simulink model "tearthtest"  (R2018b)
settings: Solver=ode45  StartTime=0.0  StopTime=365*24*3600  RelTol=1e-3  EnableMultiTasking=on
settings Model: Creator=drhf  LastModifiedBy=drhf
settings DataIOCC: LimitDataPoints=on  SaveFormat=Array  SignalLoggingSaveFormat=ModelDataLogs
settings OptimizationCC: ExpressionDepthLimit=2147483647  LifeSpan=inf
settings DebuggingCC: UnderspecifiedInitializationDetection=Classic  MergeDetectMultiDrivingBlocksExec=none  SolverPrmCheckMsg=warning  FcnCallInpInsideContextMsg=warning  StateNameClashWarn=warning  SFUnexpectedBacktrackingDiag=warning  SFNoUnconditionalDefaultTransitionDiag=warning  SFExecutionAtInitializationDiag=none
settings HardwareCC: ProdBitPerPointer=32  ProdBitPerSizeT=32  ProdBitPerPtrDiffT=32  ProdLargestAtomicFloat=None  ProdIntDivRoundTo=Undefined  ProdEndianess=Unspecified  ProdWordSize=32  ProdHWDeviceType=32-bit Generic
settings ModelReferenceCC: PropagateSignalLabelsOutOfModel=off
settings SFSimCC: SimUseLocalCustomCode=off
settings RTWCC: RTWUseLocalCustomCode=off
settings CodeAppCC: StateflowObjectComments=on
settings GRTTargetCC: TargetLangStandard=C89/C90 (ANSI)  GeneratePreprocessorConditionals=Disable all  CombineOutputUpdateFcns=off  GRTInterface=on
settings ConfigComp: CovMetricSettings=dw  CovHtmlReporting=on  CovSaveCumulativeToWorkspaceVar=on  CovSaveSingleToWorkspaceVar=on  CovExternalEMLEnable=off

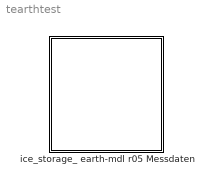
== system tearthtest ==
  ice_storage_ earth-mdl r05 Messdaten : Subsystem  mask(simple water storage){vol=10, l_solar=30*3, l_hp=8*40, f_ice=0.075, t_ini=0, z=3.32-0.12, h=7, dearth=1, Tmeanoutside=11, deltathetae=9.3, Tmeaninside=5, deltathetai=15, tshift=319 %+8760/2 %to get the right behaviour!, cond_ground=5, cp_ground=800, rho_ground=2500}
      mask prompts: vol "volume [m³]"; l_solar "length of solar heat exchanger [m]"; l_hp "length of HP heat exchanger [m]"; f_ice "Initial fraction of ice (0..1)"; t_ini "Initial Temperatur (only if fraction ice = 0) [°C]"; z "depth of baseplate from upper surface [m]"; h "height of ice storage [m]"; dearth "thickness of surrounding earth layer [m]"; Tmeanoutside "mean outside temperature over one year [°C]"; deltathetae "amplitude of monthly outside temperatures [°C]"; Tmeaninside "mean inside temperature over one year [°C]"; deltathetai "amplitude of monthly mean inside temperature [°C]"; tshift "time shift where external temperature sine-curve shows a minimum [h]"; cond_ground "conductivity of ground [W/(m*K)]"; cp_ground "capacity of ground [J/(kg*K)]"; rho_ground "density of ground [kg/m^3]"
      mask help: multinode water storage
      mask init:
      | f_ice = min(1, max(0, f_ice));
      | h_ini = (1-f_ice)*335e3;
      | if f_ice == 0 
      |     h_ini = h_ini + 4182*t_ini;
      | end
      | %Durchmesser Eisspeicher [m]
      | D_tank = 2.7;
      | %Höhe Eisspeicher [m]
      | h_tank = 2.3;
      | %Grundfläche [m^2]
      | A = pi*(D_tank/2.)^2;
      | %Umfang [m]
      | P = D_tank*pi;
      | %charakteristisches Bodenmass [m]
      | B = A/(0.5*P);
      | %Wärmewiderstand Boden & Wand [m^2*K/W]
      | Rbtot = 0.12/1.330;
      | Rwtot = 0.1/1.330;
      | %Wanddicke [m]
      | w = 0.1;
      | %wirksame Dicke Boden & Wand [m]
      | dt = w + cond_ground*Rbtot;
      | dw = cond_ground*Rwtot;
      | %abstand der mitte der wandfläche zur oberfläche [m]
      | ztilde = z-(0.5*h);
      | %anzahl stunden pro jahr
      | t0 = 8760;
      | %thermische eindringtiefe
      | delta_grd = sqrt((t0*3600*cond_ground)/(pi*rho_ground*cp_ground));
      | 
      | %U-Wert Erdschicht [W/m^2K]
      | U_earth = cond_ground/dearth;
      | %Oberfläche Erdschicht [m^2]
      | A_earth = ((D_tank+2*dearth)/2)^2*pi + (D_tank+2*dearth)*pi*(h_tank+dearth);
      | %Volumen Erdschicht [m^3]
      | V_earth = ((D_tank+2*dearth)/2)^2*pi*(h_tank+dearth) - (D_tank/2)^2*pi*h_tank;
      | %U*A tank
      | UA_tank = (D_tank/2)^2*pi/(0.12/1.330) + D_tank*pi*h_tank/(0.1/1.330);
      | 
      | 
      | tshift*2*pi/(365*24) 
      | ztilde/delta_grd
      mask Help: eval('man(''storage'')')
      mask Display: plot(0,0,100,100,[20,30,40,50,60,70,70,60,50,40,30,20,20],[70,90,84,84,90,70,20,13,10,10,13,20,70],[60,50,40,30],[90,95,95,90],[70,60,50,40,30,20],[70,64,60,60,64,70],[45,45],[20,50],[56,35],[35,35],[53,37],[26,44],[53,37],[44,26],[48,45,42],[46,43,46],[54,51,54],[33,35,38],[48,45,42],[24,28,23],[37,40,37],[32,35,38])

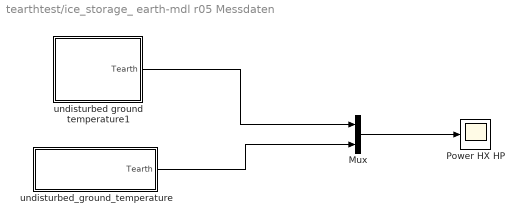
== system tearthtest/ice_storage_ earth-mdl r05 Messdaten ==
  Mux : Mux  Inputs=2
  Power HX HP : Scope
  undisturbed ground temperature1 : Subsystem
  undisturbed_ground_temperature : Subsystem  mask{Tmeanoutside=Tmeanoutside, deltathetae=deltathetae, tshift=tshift, cond_ground=cond_ground, rho_ground=rho_ground, cp_ground=cp_ground}
      mask prompts: Tmeanoutside "mean outside temperature over one year [°C]"; deltathetae "amplitude of monthly outside temperatures [°C]"; tshift "time shift where external temperature sine-curve shows a minimum [h]"; cond_ground "soil conductivity"; rho_ground "soil density"; cp_ground "soil heat capacity"
      mask init:
      | %thermische eindringtiefe
      | delta_grd = sqrt((8760*3600*cond_ground)/(pi*rho_ground*cp_ground));
  wires:
  undisturbed ground temperature1/1(Tearth) -> Mux/1
  Mux/1 -> Power HX HP/1
  undisturbed_ground_temperature/1(Tearth) -> Mux/2

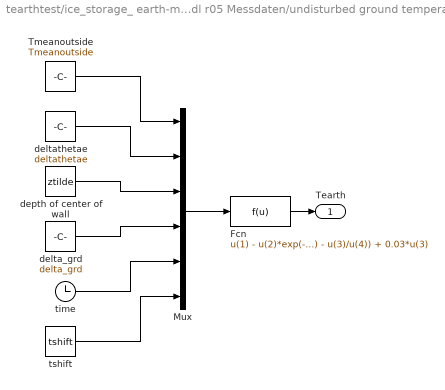
== system tearthtest/ice_storage_ earth-mdl r05 Messdaten/undisturbed ground temperature1 ==
  Fcn : Fcn  Expr=u(1) - u(2)*exp(-u(3)/u(4))*cos(2*pi*(u(5)-u(6)*3600)/(365*24*3600) - u(3)/u(4)) + 0.03*u(3)
  Mux : Mux  Inputs=6
  Tmeanoutside : Constant  Value=Tmeanoutside
  delta_grd : Constant  Value=delta_grd
  deltathetae : Constant  Value=deltathetae
  depth of center of wall : Constant  Value=ztilde
  time : Clock
  tshift : Constant  Value=tshift
  Tearth : Outport
  wires:
  Fcn/1 -> Tearth/1
  Mux/1 -> Fcn/1
  tshift/1 -> Mux/6
  time/1 -> Mux/5
  delta_grd/1 -> Mux/4
  depth of center of wall/1 -> Mux/3
  deltathetae/1 -> Mux/2
  Tmeanoutside/1 -> Mux/1

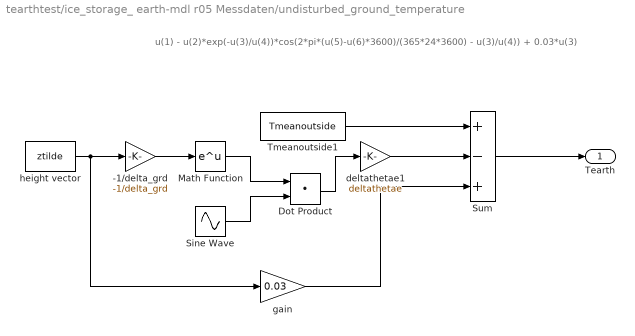
== system tearthtest/ice_storage_ earth-mdl r05 Messdaten/undisturbed_ground_temperature ==
  note: u(1) - u(2)*exp(-u(3)/u(4))*cos(2*pi*(u(5)-u(6)*3600)/(365*24*3600) - u(3)/u(4)) + 0.03*u(3)
  -1/delta_grd : Gain  Gain=-1/delta_grd
  Dot Product : DotProduct  InputSameDT=on  OutDataTypeStr=Inherit: Inherit via internal rule
  Math Function : Math  SaturateOnIntegerOverflow=on
  Sine Wave : Sin  Frequency=2*pi/(365*24*3600)  Phase=pi/2 - tshift*2*pi/(365*24) - ztilde/delta_grd  SampleTime=0
  Sum : Sum  Inputs=+-+
  Tmeanoutside1 : Constant  Value=Tmeanoutside
  deltathetae1 : Gain  Gain=deltathetae
  gain : Gain  Gain=0.03
  height vector : Constant  Value=ztilde
  Tearth : Outport
  wires:
  height vector/1 -> -1/delta_grd/1, gain/1
  -1/delta_grd/1 -> Math Function/1
  deltathetae1/1 -> Sum/2
  Math Function/1 -> Dot Product/1
  Sine Wave/1 -> Dot Product/2
  Dot Product/1 -> deltathetae1/1
  gain/1 -> Sum/3
  Sum/1 -> Tearth/1
  Tmeanoutside1/1 -> Sum/1
